simulink model "WMMSupportingForcesGP2020a"  (R2020a)
settings: Solver=ode23t  StartTime=0.0  StopTime=inf  FixedStep=.001  RelTol=1e-3  AbsTol=1e-3
InitFcn:
  | InitializeSimulationGP
  | SimulationParametersGP
values from neighbouring files (symbols this model uses):
  B11_r_B11C = [0.23805608; 0.13201777; 0]    [InitializeSimulationGP.m]
  B11_r_B11Tc1 = [L11; 0; 0]    [InitializeSimulationGP.m]
  B11_Rot_Tc1 = eye(3)    [InitializeSimulationGP.m]
  B11cI = [0.28426000 -0.06487287 0;         -0.06487287  0.54237481 0;                   0  0          0.67891020]    [InitializeSimulationGP.m]
  B12_r_B12C = [0.60504569; 0.27199376; 0.00002484]    [InitializeSimulationGP.m]
  B12_r_B12Tc2 = [L12;0;0]    [InitializeSimulationGP.m]
  B12_Rot_Tc2 = eye(3)    [InitializeSimulationGP.m]
  B12cI = [1.18803886 -2.36786418 0.00280315;          -2.36786418 6.31493281 0.00022322;           0.00280315 0.00022322 7.40915161]    [InitializeSimulationGP.m]
  B31_r_B31C = [0.35781210 0 0]    [InitializeSimulationGP.m]
  B31_Rot_B41 = eye(3)    [InitializeSimulationGP.m]
  B31cI = diag([0.03150902 0.90735702 0.90763033])    [InitializeSimulationGP.m]
  B32_r_B32C = [0.35781210 0 0]    [InitializeSimulationGP.m]
  B32_Rot_B42 = eye(3)    [InitializeSimulationGP.m]
  B32cI = diag([0.03150902 0.90735702 0.90763033])    [InitializeSimulationGP.m]
  B41_r_B41C = [0.55785997 0 0]    [InitializeSimulationGP.m]
  B41_r_B41Tc1 = [lc1;0;0]    [InitializeSimulationGP.m]
  B41cI = diag([0.00370720 0.55759812 0.55785997])    [InitializeSimulationGP.m]
  B42_r_B42C = [0.55785997 0 0]    [InitializeSimulationGP.m]
  B42_r_B42Tc2 = [lc2; 0; 0]    [InitializeSimulationGP.m]
  B42cI = diag([0.00370720 0.55759812 0.55785997])    [InitializeSimulationGP.m]
  B52_r_B52C = [0 0 0.56802906]    [InitializeSimulationGP.m]
  B52_r_B52P32 = [lc3; 0; 0]    [InitializeSimulationGP.m]
  B52_Rot_P32 = eye(3)    [InitializeSimulationGP.m]
  B52cI = diag([0.91789884, 0.91790043, 0.00091463])    [InitializeSimulationGP.m]
  Bc1_r_Bc1B11 = [L1; 0; 0]    [InitializeSimulationGP.m]
  Bc1_r_Bc1B31 = [0;0;0]    [InitializeSimulationGP.m]
  Bc1_r_Bc1C = [0.14178771; 0.16555780; 0]    [InitializeSimulationGP.m]
  Bc1_V = [0;0;0;0;0;0]    [InitializeSimulationGP.m]
  Bc1cI = [+5.892211080 +5.476111360 -0.000019630;          +5.476111360 +28.66965601 -0.000024550;          -0.000019630 -0.000024550 +29.78955950]    [InitializeSimulationGP.m]
  Bc2_r_Bc2B12 = [L2;0;0]    [InitializeSimulationGP.m]
  Bc2_r_Bc2B32 = [0;0;0]    [InitializeSimulationGP.m]
  Bc2_r_Bc2C = [0.54319901; 0.10543875; 0]    [InitializeSimulationGP.m]
  Bc2cI = [0.48071390 0.52924041 0;          0.52924041 5.80912352 0;              0      0          5.97255351]    [InitializeSimulationGP.m]
  BC_r_BCBM = [xCA; yCA; zCA]    [SimulationParametersGP.m]
  BC_Rot_BM = eye(3)    [SimulationParametersGP.m]
  BCI = diag([100 1200 1000])    [SimulationParametersGP.m]
  beta1 = atan2d(374.261,935)*pi/180    [InitializeSimulationGP.m]
  beta2 = atan2d(45.757,373.313)*pi/180    [InitializeSimulationGP.m]
  beta3 = atan2d(139.50,1132.19)*pi/180    [InitializeSimulationGP.m]
  beta4 = atan2d(88.061,296.198)*pi/180    [InitializeSimulationGP.m]
  betaGround = 1e6    (= 1000000)    [SimulationParametersGP.m]
  BFL = 0.05    [SimulationParametersGP.m]
  BFR = 0.05    [SimulationParametersGP.m]
  BM_r_BMBMp = [0;0;0]    [SimulationParametersGP.m]
  BM_Rot_BMp = [cos(gamma) -sin(gamma) 0; sin(gamma) cos(gamma) 0; 0 0 1]    [SimulationParametersGP.m]
  BMp_r_BMpBc1 = [0.185;0;0.205]    [InitializeSimulationGP.m]
  BMp_Rot_Bc1 = [cos(alpha1) -sin(alpha1)  0;                  0            0       -1;                sin(alpha1)  cos(alpha1)  0]    [InitializeSimulationGP.m]
  BRL = 0.05    [SimulationParametersGP.m]
  BRR = 0.05    [SimulationParametersGP.m]
  cc = 0.0    (= 0)    [SimulationParametersGP.m]
  D22F = [0;0;0;0;0;0]    [InitializeSimulationGP.m]
  dT = 0.01    [SimulationParametersGP.m]
  g0 = 9.8066    [SimulationParametersGP.m]
  ground_stiffness = 1e8    (= 100000000)    [SimulationParametersGP.m]
  l1 = 1.15-cc    (= 1.15)    [SimulationParametersGP.m]
  L1 = 1.0071227324212    (= 1.00712273242)    [InitializeSimulationGP.m]
  L11 = 0.37610632101293    (= 0.376106321013)    [InitializeSimulationGP.m]
  L12 = 0.30901132665325    (= 0.309011326653)    [InitializeSimulationGP.m]
  l2 = 1.15+cc    (= 1.15)    [SimulationParametersGP.m]
  L2 = 1.132185817991    (= 1.13218581799)    [InitializeSimulationGP.m]
  lc1 = 0.745    [InitializeSimulationGP.m]
  lc2 = 0.745    [InitializeSimulationGP.m]
  mB11 = 25.52660174    [InitializeSimulationGP.m]
  mB12 = 33.92850233    [InitializeSimulationGP.m]
  mB31 = 17.36281648    [InitializeSimulationGP.m]
  mB32 = 17.36281648    [InitializeSimulationGP.m]
  mB41 = 10.34519231    [InitializeSimulationGP.m]
  mB42 = 10.34519231    [InitializeSimulationGP.m]
  mB52 = 6.73059863    [InitializeSimulationGP.m]
  mBC = 2200    [SimulationParametersGP.m]
  mBc1 = 307.29601379    [InitializeSimulationGP.m]
  mBc2 = 54.58702836    [InitializeSimulationGP.m]
  mFL = 60    [SimulationParametersGP.m]
  mFR = 60    [SimulationParametersGP.m]
  mP22 = 9.26136143    [InitializeSimulationGP.m]
  mP32 = 570.18877059    [InitializeSimulationGP.m]
  mRR = 60    [SimulationParametersGP.m]
  mw = mFL    (= 60)    [SimulationParametersGP.m]
  P22_r_P22C = [0.62192523 0 0]    [InitializeSimulationGP.m]
  P22_Rot_B52 = eye(3)    [InitializeSimulationGP.m]
  P22cI = diag([0.00662754, 1.48387017, 1.48398069])    [InitializeSimulationGP.m]
  P32_r_P32C = [0.25466704; -0.13034397; -0.01302248]    [InitializeSimulationGP.m]
  P32_r_P32D22 = [0.40499744871392; -0.13130517281345; -0.013385243295654]    [InitializeSimulationGP.m]
  P32_Rot_D22 = [1 0 0;              0 0.9707729441837 0.23999977258512;              0 -0.23999977258512 0.9707729441837]    [InitializeSimulationGP.m]
  P32cI = [46.81220713 0.38607676 -0.00453819;          0.38607676 71.92201786 -1.14320993;          -0.00453819 -1.14320993 67.38128576]    [InitializeSimulationGP.m]
  R0FL = 0.35    [SimulationParametersGP.m]
  R0FR = 0.35    [SimulationParametersGP.m]
  R0RL = 0.35    [SimulationParametersGP.m]
  R0RR = 0.35    [SimulationParametersGP.m]
  Rw = R0FL    (= 0.35)    [SimulationParametersGP.m]
  Tc1_r_Tc1Bc2 = [0.098495302558553; 0.01838181329939; 0]    [InitializeSimulationGP.m]
  Tc1_Rot_Bc2 = [cos(alpha2) -sin(alpha2) 0;                sin(alpha2)  cos(alpha2) 0;                0            0           1]    [InitializeSimulationGP.m]
  Tc2_r_Tc2P22 = [-0.048858374920227;0.36587359346146;0.035276938723102]    [InitializeSimulationGP.m]
  Tc2_Rot_P22 = [0.95853460763586 -0.27664713597974  0.0683942111482;                0.28497614981675  0.93051946315663 -0.23004808784757;                0                 0.23999977258511  0.9707729441837]    [InitializeSimulationGP.m]
  Th1A = 10*pi/180    (= 0.174532925199)    [InitializeSimulationGP.m]
  Th1B = 20*pi/180    (= 0.349065850399)    [InitializeSimulationGP.m]
  Th1f = 1    [InitializeSimulationGP.m]
  Th2A = 15*pi/180    (= 0.261799387799)    [InitializeSimulationGP.m]
  Th2B = -70*pi/180    (= -1.2217304764)    [InitializeSimulationGP.m]
  Th2f = 2    [InitializeSimulationGP.m]
  w = wFL    (= 0.875)    [SimulationParametersGP.m]
  W_r_WBc1 = [0.185;0;0.205]    [InitializeSimulationGP.m]
  W_Rot_Bc1 = [cos(alpha1) -sin(alpha1)  0;                  0            0       -1;                sin(alpha1)  cos(alpha1)  0]    [InitializeSimulationGP.m]
  x10 = 0.83    [InitializeSimulationGP.m]
  x20 = 0.83    [InitializeSimulationGP.m]
  x3A = 0.2    [InitializeSimulationGP.m]
  x3B = 0.3    [InitializeSimulationGP.m]
  x3f = 1    [InitializeSimulationGP.m]
  xCA = 0.5    [SimulationParametersGP.m]
  xf = [1;0;0;0;0;0]    [InitializeSimulationGP.m]
  yCA = 0    [SimulationParametersGP.m]
  zC = 0.45    [SimulationParametersGP.m]
  zCA = .25    (= 0.25)    [SimulationParametersGP.m]
  ztau = [0;0;0;0;0;1]    [InitializeSimulationGP.m]
undefined symbols (not defined in the file or in its folder): alphaFL_meas, alphaFR_meas, alphaRL_meas, alphaRR_meas, B11_V, B11Ftot, B12_U_Tc2, B12_V, B12Ftot, B31_r_B31B41, B31_V, B31FTot, B32_r_B32B42, B32_U_B42, B32_V, B32FTot, B41_V, B41FTot, B42_Rot_Tc2, B42_U_Tc2, B42_V, B42FTot, B52_U_P32, B52_V, B52Ftot, Bc1Tot, Bc2_Rot_B12, Bc2_Rot_B32, Bc2_U_B12, Bc2_U_B32, Bc2_V, Bc2Tot, betaC_meas, D22_V, deltaFL_cmd, deltaFL_meas, deltaFR_cmd, deltaFR_meas, deltaRL_cmd, deltaRL_meas, deltaRR_cmd, deltaRR_meas, dOmegaFL_meas, dOmegaFR_meas, dOmegaRL_meas, dOmegaRR_meas, dPsi_meas, dq1, dq11, dq12, dq2, dq21, dq22, dx1, dx2, Floor, FTot_S1, FTot_S2P, FTot_S2R, FzFL ... (+63)
libraries: sm_lib x94, nesl_utility x63, simulink x5
(part 4 of 11)

== system WMMSupportingForcesGP2020a/Mobile Manipulator in Simscape/Hydraulic manipulator, Simscape ==
  note: Hydraulic manipulator in Simscape
  note: Linear hydraulic actuator forces
  Theta1 [rad] : Inport
  Theta2 [rad] : Inport  Port=2
  x3[m] : Inport  Port=3
  Base : Subsystem
      settings: PortSchema="{\"entries\":[{\"content\":{\"sides\":[{\"content\":{\"connectorIds\":[\"In1\",\"LConn1\"]},\"type\":\"ConnectorPlacement.EquallySpacedRectSide\",\"uuid\":\"74e7f3c6-cbce-4102-a556-47a2132f5eea\"},{\"content\":{\"connectorIds\":[\"RConn1\",\"RConn2\"],\"side\":\"RIGHT\"},\"type\":\"ConnectorPlacement.EquallySpacedRectSide\",\"uuid\":\"9dc74751-c8ff-4cb6-874a-dcd58e00de96\"},{\"content\":{\"connectorIds\":[\"LConn2\"],\"side\":\"TOP\"},\"type\":\"ConnectorPlacement.EquallySpacedRectSide\",\"uuid\":\"06e145de-a8a9-4531-940d-434d89c78f5b\"}]},\"type\":\"ConnectorPlacement.EquallySpacedConnector\",\"uuid\":\"f796a1f4-9531-411f-8f55-fdef488b8a52\"}],\"packageUris\":[\"http://schema.mathworks.com/mf0/Connector/R2020b\"],\"version\":\"1.0\"}"
  Bus Creator1 : BusCreator  Inputs=3
  Connection Label1 : ConnectionLabel  Label=BMp
  Connection Label11 : ConnectionLabel  Label=B12
  Connection Label12 : ConnectionLabel  Label=B52
  Connection Label14 : ConnectionLabel  Label=Bc1
  Connection Label15 : ConnectionLabel  Label=Tc2
  Connection Label16 : ConnectionLabel  Label=D22
  Connection Label29 : ConnectionLabel  Label=P22
  Connection Label3 : ConnectionLabel  Label=Tc1
  Connection Label32 : ConnectionLabel  Label=P32
  Connection Label4 : ConnectionLabel  Label=B11
  Connection Label5 : ConnectionLabel  Label=Bc2
  Connection Label6 : ConnectionLabel  Label=B31
  Connection Label7 : ConnectionLabel  Label=B42
  Connection Label8 : ConnectionLabel  Label=B32
  Connection Label9 : ConnectionLabel  Label=B41
  EndMassObject : Subsystem
      settings: PortSchema="{\"entries\":[{\"content\":{\"sides\":[{\"content\":{\"connectorIds\":[]},\"type\":\"ConnectorPlacement.EquallySpacedRectSide\",\"uuid\":\"c1652833-a888-40a4-a60e-17be9708feae\"},{\"content\":{\"connectorIds\":[],\"side\":\"RIGHT\"},\"type\":\"ConnectorPlacement.EquallySpacedRectSide\",\"uuid\":\"55671429-adc4-418e-b6f5-c624f049c776\"},{\"content\":{\"connectorIds\":[\"LConn1\",\"LConn2\"],\"side\":\"TOP\"},\"type\":\"ConnectorPlacement.EquallySpacedRectSide\",\"uuid\":\"549e793d-1b28-4f93-9706-f4524b8bc4e2\"}]},\"type\":\"ConnectorPlacement.EquallySpacedConnector\",\"uuid\":\"9a6e434f-5824-411f-a3a4-9b8ec603a501\"}],\"packageUris\":[\"http://schema.mathworks.com/mf0/Connector/R2020b\"],\"version\":\"1.0\"}"
  LiftCylinderAndLiftPiston : Subsystem
      settings: PortSchema="{\"entries\":[{\"content\":{\"sides\":[{\"content\":{\"connectorIds\":[]},\"type\":\"ConnectorPlacement.EquallySpacedRectSide\",\"uuid\":\"a609877c-275e-4024-96c6-67831631fbf9\"},{\"content\":{\"connectorIds\":[\"Out1\"],\"side\":\"RIGHT\"},\"type\":\"ConnectorPlacement.EquallySpacedRectSide\",\"uuid\":\"b747ace3-04d7-42f4-87a7-c62fd6093e0d\"},{\"content\":{\"connectorIds\":[\"LConn1\",\"LConn2\"],\"side\":\"TOP\"},\"type\":\"ConnectorPlacement.EquallySpacedRectSide\",\"uuid\":\"5f9db8d6-814e-4333-b197-0e9dcf847d3e\"},{\"content\":{\"connectorIds\":[\"RConn1\",\"RConn2\"],\"side\":\"BOTTOM\"},\"type\":\"ConnectorPlacement.EquallySpacedRectSide\",\"uuid\":\"d1d564c3-4146-4330-9936-8dd25e0cb4bf\"}]},\"type\":\"ConnectorPlacement.EquallySpacedConnector\",\"uuid\":\"d00f43c3-717c-4aa5-b919-dd57ad6708f7\"}],\"packageUris\":[\"http://schema.mathworks.com/mf0/Connector/R2020b\"],\"version\":\"1.0\"}"
  LiftLink : Subsystem
      settings: PortSchema="{\"entries\":[{\"content\":{\"sides\":[{\"content\":{\"connectorIds\":[\"LConn1\",\"LConn2\"]},\"type\":\"ConnectorPlacement.EquallySpacedRectSide\",\"uuid\":\"50668ed3-3246-41c6-a320-c5b34ebd86b6\"},{\"content\":{\"connectorIds\":[\"In1\",\"RConn1\"],\"side\":\"RIGHT\"},\"type\":\"ConnectorPlacement.EquallySpacedRectSide\",\"uuid\":\"d76ddc23-e4dc-4bdf-9e15-3eadac6cf1e2\"},{\"content\":{\"connectorIds\":[\"LConn3\"],\"side\":\"TOP\"},\"type\":\"ConnectorPlacement.EquallySpacedRectSide\",\"uuid\":\"5458eee7-805c-4d74-888c-3f811d80880c\"},{\"content\":{\"connectorIds\":[\"RConn2\",\"RConn3\",\"RConn4\"],\"side\":\"BOTTOM\"},\"type\":\"ConnectorPlacement.EquallySpacedRectSide\",\"uuid\":\"6f630415-b321-44c9-a6f9-9daa6b5086dd\"}]},\"type\":\"ConnectorPlacement.EquallySpacedConnector\",\"uuid\":\"adbb0eba-5908-47e0-8cde-3ca3a2901b66\"}],\"packageUris\":[\"http://schema.mathworks.com/mf0/Connector/R2020b\"],\"version\":\"1.0\"}"
  PrismaticJointCylinderAndPiston : Subsystem
      settings: PortSchema="{\"entries\":[{\"content\":{\"sides\":[{\"content\":{\"connectorIds\":[\"In1\"]},\"type\":\"ConnectorPlacement.EquallySpacedRectSide\",\"uuid\":\"002196eb-b81c-4ad4-9df1-33c4ef5d5c77\"},{\"content\":{\"connectorIds\":[\"Out1\"],\"side\":\"RIGHT\"},\"type\":\"ConnectorPlacement.EquallySpacedRectSide\",\"uuid\":\"e0d61efe-ea5d-4756-bea5-1d107b09975a\"},{\"content\":{\"connectorIds\":[],\"side\":\"TOP\"},\"type\":\"ConnectorPlacement.EquallySpacedRectSide\",\"uuid\":\"1a952641-c922-4f91-9854-1cf1d6e715db\"},{\"content\":{\"connectorIds\":[\"RConn1\",\"RConn2\",\"RConn3\"],\"side\":\"BOTTOM\"},\"type\":\"ConnectorPlacement.EquallySpacedRectSide\",\"uuid\":\"13c3128f-85d9-4df5-9ae2-f45a9cb5a20e\"}]},\"type\":\"ConnectorPlacement.EquallySpacedConnector\",\"uuid\":\"7bd12321-8448-494e-b8ce-fe2f63fec7f7\"}],\"packageUris\":[\"http://schema.mathworks.com/mf0/Connector/R2020b\"],\"version\":\"1.0\"}"
  TilitLink : Subsystem
      settings: PortSchema="{\"entries\":[{\"content\":{\"sides\":[{\"content\":{\"connectorIds\":[]},\"type\":\"ConnectorPlacement.EquallySpacedRectSide\",\"uuid\":\"3124f0ed-3daa-4e61-aa81-877c0a0fd3a0\"},{\"content\":{\"connectorIds\":[\"RConn1\"],\"side\":\"RIGHT\"},\"type\":\"ConnectorPlacement.EquallySpacedRectSide\",\"uuid\":\"bc27bd78-7de5-476c-8b4b-17e2ed4c2476\"},{\"content\":{\"connectorIds\":[\"LConn1\",\"LConn2\",\"LConn3\",\"LConn4\"],\"side\":\"TOP\"},\"type\":\"ConnectorPlacement.EquallySpacedRectSide\",\"uuid\":\"46b542cf-bb62-4410-9418-b726c84ee3f9\"}]},\"type\":\"ConnectorPlacement.EquallySpacedConnector\",\"uuid\":\"3938a7f2-fa69-42c9-abcf-1c8c25e9b66f\"}],\"packageUris\":[\"http://schema.mathworks.com/mf0/Connector/R2020b\"],\"version\":\"1.0\"}"
  TiltCylinderAndTiltPiston : Subsystem
      settings: PortSchema="{\"entries\":[{\"content\":{\"sides\":[{\"content\":{\"connectorIds\":[]},\"type\":\"ConnectorPlacement.EquallySpacedRectSide\",\"uuid\":\"a609877c-275e-4024-96c6-67831631fbf9\"},{\"content\":{\"connectorIds\":[\"Out1\"],\"side\":\"RIGHT\"},\"type\":\"ConnectorPlacement.EquallySpacedRectSide\",\"uuid\":\"b747ace3-04d7-42f4-87a7-c62fd6093e0d\"},{\"content\":{\"connectorIds\":[\"LConn1\",\"LConn2\"],\"side\":\"TOP\"},\"type\":\"ConnectorPlacement.EquallySpacedRectSide\",\"uuid\":\"5f9db8d6-814e-4333-b197-0e9dcf847d3e\"},{\"content\":{\"connectorIds\":[\"RConn1\",\"RConn2\"],\"side\":\"BOTTOM\"},\"type\":\"ConnectorPlacement.EquallySpacedRectSide\",\"uuid\":\"d1d564c3-4146-4330-9936-8dd25e0cb4bf\"}]},\"type\":\"ConnectorPlacement.EquallySpacedConnector\",\"uuid\":\"d00f43c3-717c-4aa5-b919-dd57ad6708f7\"}],\"packageUris\":[\"http://schema.mathworks.com/mf0/Connector/R2020b\"],\"version\":\"1.0\"}"
  BMp : PMIOPort  Side=Left
  fcx_SS : Outport
  wires:
  LiftCylinderAndLiftPiston/1(fc1) -> [fc1]
  TiltCylinderAndTiltPiston/1(fc2) -> [fc2]
  x3[m]/1 -> PrismaticJointCylinderAndPiston/1(x3)
  PrismaticJointCylinderAndPiston/1(fc3) -> [fc3]
  Theta1 [rad]/1 -> Base/1(Theta1[rad])
  Theta2 [rad]/1 -> LiftLink/1(Theta2[rad])
  [fc1] -> Bus Creator1/1  "fc1_SS"
  [fc2] -> Bus Creator1/2  "fc2_SS"
  [fc3] -> Bus Creator1/3  "fc3_SS"
  Bus Creator1/1 -> fcx_SS/1
  connections:
  BMp/RConn1 -- Base/LConn1 -- Connection Label1/LConn1
  LiftLink/LConn1 -- TiltCylinderAndTiltPiston/RConn1
  LiftLink/LConn2 -- TilitLink/RConn1
  TiltCylinderAndTiltPiston/RConn2 -- TilitLink/LConn4
  LiftCylinderAndLiftPiston/RConn2 -- LiftLink/LConn3
  Base/RConn2 -- LiftLink/RConn1
  LiftCylinderAndLiftPiston/RConn1 -- Base/RConn1
  LiftLink/RConn4 -- Connection Label3/LConn1
  Connection Label4/LConn1 -- LiftLink/RConn3
  Connection Label5/LConn1 -- LiftLink/RConn2
  Connection Label6/LConn1 -- LiftCylinderAndLiftPiston/LConn1
  Connection Label9/LConn1 -- LiftCylinderAndLiftPiston/LConn2
  Connection Label7/LConn1 -- TiltCylinderAndTiltPiston/LConn2
  Connection Label8/LConn1 -- TiltCylinderAndTiltPiston/LConn1
  Connection Label11/LConn1 -- TilitLink/LConn3
  Connection Label15/LConn1 -- TilitLink/LConn2
  Connection Label16/LConn1 -- EndMassObject/LConn2
  Connection Label14/LConn1 -- Base/LConn2
  Connection Label12/LConn1 -- PrismaticJointCylinderAndPiston/RConn3
  PrismaticJointCylinderAndPiston/RConn1 -- Connection Label29/LConn1 -- TilitLink/LConn1
  PrismaticJointCylinderAndPiston/RConn2 -- EndMassObject/LConn1 -- Connection Label32/LConn1

== system WMMSupportingForcesGP2020a/Mobile Manipulator in Simscape/SteeringFL ==
  deltaFL_cmd : Inport
  PS-Simulink Converter : nesl_utility/PS-Simulink Converter  PhysicalDomain=network_engine_domain  SubClassName=ps_output  LeftPortType=input  RightPortType=output  PseudoPeriodic=off  Frequencies=[]  Unit=inherit  AffineConversion=off
      settings: SourceProductBaseCode=PW,SS
  Revolute Joint2 : sm_lib/Joints/Revolute Joint  JointMode=Normal  SenseConstraintForce=off  SenseConstraintForceX=off  SenseConstraintForceY=off  SenseConstraintForceZ=off  SenseConstraintTorque=off  SenseConstraintTorqueX=off  SenseConstraintTorqueY=off  SenseConstraintTorqueZ=off  SenseTotalForce=off  SenseTotalForceX=off  SenseTotalForceY=off  SenseTotalForceZ=off  SenseTotalTorque=off  SenseTotalTorqueX=off  SenseTotalTorqueY=off  SenseTotalTorqueZ=off  CompositeWrenchDir=FollowerOnBase  CompositeWrenchFrame=BaseFrame  EquilibriumPosition=0  EquilibriumPositionUnits=rad  SpringStiffness=0  SpringStiffnessUnits=N*m/rad  DampingCoefficient=.0001  DampingCoefficientUnits=N*m/(rad/s)  TorqueActuationMode=ComputedTorque  MotionActuationMode=InputMotion  SensePosition=on  SenseVelocity=off  SenseAcceleration=off  SenseTorqueForce=off  SenseLowerLimitTorqueForce=off  SenseUpperLimitTorqueForce=off  LowerLimitSpecify=off  LowerLimitBound=-90  LowerLimitBoundUnits=deg  LowerLimitStiffness=1e4  LowerLimitStiffnessUnits=N*m/deg  LowerLimitDamping=10  LowerLimitDampingUnits=N*m/(deg/s)  LowerLimitTransitionRegionWidth=0.1  LowerLimitTransitionRegionWidthUnits=deg  UpperLimitSpecify=off  UpperLimitBound=90  UpperLimitBoundUnits=deg  UpperLimitStiffness=1e4  UpperLimitStiffnessUnits=N*m/deg  UpperLimitDamping=10  UpperLimitDampingUnits=N*m/(deg/s)  UpperLimitTransitionRegionWidth=0.1  UpperLimitTransitionRegionWidthUnits=deg  PositionTargetSpecify=off  PositionTargetPriority=High  PositionTargetValue=0  PositionTargetValueUnits=deg  VelocityTargetSpecify=off  VelocityTargetPriority=High  VelocityTargetValue=0  VelocityTargetValueUnits=deg/s
  Simulink-PS Converter7 : nesl_utility/Simulink-PS Converter  PhysicalDomain=network_engine_domain  SubClassName=ps_input  LeftPortType=input  RightPortType=output  PseudoPeriodic=off  Frequencies=[]  NoiseDistribution=none  NoiseParameters=[]  Unit=rad  AffineConversion=off  FilteringAndDerivatives=filter  SimscapeFilterOrder=2  InputFilterTimeConstant=0.001  UdotUserProvided=0
      settings: SourceProductBaseCode=PW,SS
  WFL : PMIOPort  Side=Left
  CFL : PMIOPort  Port=2  Side=Right
  deltaFL_meas : Outport
  wires:
  deltaFL_cmd/1 -> Simulink-PS Converter7/1
  PS-Simulink Converter/1 -> deltaFL_meas/1
  connections:
  Simulink-PS Converter7/RConn1 -- Revolute Joint2/LConn2
  Revolute Joint2/LConn1 -- CFL/RConn1
  Revolute Joint2/RConn1 -- WFL/RConn1
  PS-Simulink Converter/LConn1 -- Revolute Joint2/RConn2

== system WMMSupportingForcesGP2020a/Mobile Manipulator in Simscape/SteeringFR ==
  deltaFR_cmd : Inport
  PS-Simulink Converter : nesl_utility/PS-Simulink Converter  PhysicalDomain=network_engine_domain  SubClassName=ps_output  LeftPortType=input  RightPortType=output  PseudoPeriodic=off  Frequencies=[]  Unit=inherit  AffineConversion=off
      settings: SourceProductBaseCode=PW,SS
  Revolute Joint2 : sm_lib/Joints/Revolute Joint  JointMode=Normal  SenseConstraintForce=off  SenseConstraintForceX=off  SenseConstraintForceY=off  SenseConstraintForceZ=off  SenseConstraintTorque=off  SenseConstraintTorqueX=off  SenseConstraintTorqueY=off  SenseConstraintTorqueZ=off  SenseTotalForce=off  SenseTotalForceX=off  SenseTotalForceY=off  SenseTotalForceZ=off  SenseTotalTorque=off  SenseTotalTorqueX=off  SenseTotalTorqueY=off  SenseTotalTorqueZ=off  CompositeWrenchDir=FollowerOnBase  CompositeWrenchFrame=BaseFrame  EquilibriumPosition=0  EquilibriumPositionUnits=rad  SpringStiffness=0  SpringStiffnessUnits=N*m/rad  DampingCoefficient=.0001  DampingCoefficientUnits=N*m/(rad/s)  TorqueActuationMode=ComputedTorque  MotionActuationMode=InputMotion  SensePosition=on  SenseVelocity=off  SenseAcceleration=off  SenseTorqueForce=off  SenseLowerLimitTorqueForce=off  SenseUpperLimitTorqueForce=off  LowerLimitSpecify=off  LowerLimitBound=-90  LowerLimitBoundUnits=deg  LowerLimitStiffness=1e4  LowerLimitStiffnessUnits=N*m/deg  LowerLimitDamping=10  LowerLimitDampingUnits=N*m/(deg/s)  LowerLimitTransitionRegionWidth=0.1  LowerLimitTransitionRegionWidthUnits=deg  UpperLimitSpecify=off  UpperLimitBound=90  UpperLimitBoundUnits=deg  UpperLimitStiffness=1e4  UpperLimitStiffnessUnits=N*m/deg  UpperLimitDamping=10  UpperLimitDampingUnits=N*m/(deg/s)  UpperLimitTransitionRegionWidth=0.1  UpperLimitTransitionRegionWidthUnits=deg  PositionTargetSpecify=off  PositionTargetPriority=High  PositionTargetValue=0  PositionTargetValueUnits=deg  VelocityTargetSpecify=off  VelocityTargetPriority=High  VelocityTargetValue=0  VelocityTargetValueUnits=deg/s
  Simulink-PS Converter7 : nesl_utility/Simulink-PS Converter  PhysicalDomain=network_engine_domain  SubClassName=ps_input  LeftPortType=input  RightPortType=output  PseudoPeriodic=off  Frequencies=[]  NoiseDistribution=none  NoiseParameters=[]  Unit=rad  AffineConversion=off  FilteringAndDerivatives=filter  SimscapeFilterOrder=2  InputFilterTimeConstant=0.001  UdotUserProvided=0
      settings: SourceProductBaseCode=PW,SS
  WFR : PMIOPort  Side=Left
  CFR : PMIOPort  Port=2  Side=Right
  deltaFR_meas : Outport
  wires:
  deltaFR_cmd/1 -> Simulink-PS Converter7/1
  PS-Simulink Converter/1 -> deltaFR_meas/1
  connections:
  Simulink-PS Converter7/RConn1 -- Revolute Joint2/LConn2
  Revolute Joint2/LConn1 -- CFR/RConn1
  Revolute Joint2/RConn1 -- WFR/RConn1
  PS-Simulink Converter/LConn1 -- Revolute Joint2/RConn2

== system WMMSupportingForcesGP2020a/Mobile Manipulator in Simscape/SteeringRL ==
  deltaRL_cmd : Inport
  PS-Simulink Converter : nesl_utility/PS-Simulink Converter  PhysicalDomain=network_engine_domain  SubClassName=ps_output  LeftPortType=input  RightPortType=output  PseudoPeriodic=off  Frequencies=[]  Unit=inherit  AffineConversion=off
      settings: SourceProductBaseCode=PW,SS
  Revolute Joint2 : sm_lib/Joints/Revolute Joint  JointMode=Normal  SenseConstraintForce=off  SenseConstraintForceX=off  SenseConstraintForceY=off  SenseConstraintForceZ=off  SenseConstraintTorque=off  SenseConstraintTorqueX=off  SenseConstraintTorqueY=off  SenseConstraintTorqueZ=off  SenseTotalForce=off  SenseTotalForceX=off  SenseTotalForceY=off  SenseTotalForceZ=off  SenseTotalTorque=off  SenseTotalTorqueX=off  SenseTotalTorqueY=off  SenseTotalTorqueZ=off  CompositeWrenchDir=FollowerOnBase  CompositeWrenchFrame=BaseFrame  EquilibriumPosition=0  EquilibriumPositionUnits=deg  SpringStiffness=0  SpringStiffnessUnits=N*m/deg  DampingCoefficient=.0001  DampingCoefficientUnits=N*m/(deg/s)  TorqueActuationMode=ComputedTorque  MotionActuationMode=InputMotion  SensePosition=on  SenseVelocity=off  SenseAcceleration=off  SenseTorqueForce=off  SenseLowerLimitTorqueForce=off  SenseUpperLimitTorqueForce=off  LowerLimitSpecify=off  LowerLimitBound=-90  LowerLimitBoundUnits=deg  LowerLimitStiffness=1e4  LowerLimitStiffnessUnits=N*m/deg  LowerLimitDamping=10  LowerLimitDampingUnits=N*m/(deg/s)  LowerLimitTransitionRegionWidth=0.1  LowerLimitTransitionRegionWidthUnits=deg  UpperLimitSpecify=off  UpperLimitBound=90  UpperLimitBoundUnits=deg  UpperLimitStiffness=1e4  UpperLimitStiffnessUnits=N*m/deg  UpperLimitDamping=10  UpperLimitDampingUnits=N*m/(deg/s)  UpperLimitTransitionRegionWidth=0.1  UpperLimitTransitionRegionWidthUnits=deg  PositionTargetSpecify=off  PositionTargetPriority=High  PositionTargetValue=0  PositionTargetValueUnits=deg  VelocityTargetSpecify=off  VelocityTargetPriority=High  VelocityTargetValue=0  VelocityTargetValueUnits=deg/s
  Simulink-PS Converter7 : nesl_utility/Simulink-PS Converter  PhysicalDomain=network_engine_domain  SubClassName=ps_input  LeftPortType=input  RightPortType=output  PseudoPeriodic=off  Frequencies=[]  NoiseDistribution=none  NoiseParameters=[]  Unit=rad  AffineConversion=off  FilteringAndDerivatives=filter  SimscapeFilterOrder=2  InputFilterTimeConstant=0.001  UdotUserProvided=0
      settings: SourceProductBaseCode=PW,SS
  WRL : PMIOPort  Side=Left
  CRL : PMIOPort  Port=2  Side=Right
  deltaRL_meas : Outport
  wires:
  deltaRL_cmd/1 -> Simulink-PS Converter7/1
  PS-Simulink Converter/1 -> deltaRL_meas/1
  connections:
  Simulink-PS Converter7/RConn1 -- Revolute Joint2/LConn2
  Revolute Joint2/LConn1 -- CRL/RConn1
  Revolute Joint2/RConn1 -- WRL/RConn1
  PS-Simulink Converter/LConn1 -- Revolute Joint2/RConn2

== system WMMSupportingForcesGP2020a/Mobile Manipulator in Simscape/SteeringRR ==
  deltaRR_cmd : Inport
  PS-Simulink Converter : nesl_utility/PS-Simulink Converter  PhysicalDomain=network_engine_domain  SubClassName=ps_output  LeftPortType=input  RightPortType=output  PseudoPeriodic=off  Frequencies=[]  Unit=inherit  AffineConversion=off
      settings: SourceProductBaseCode=PW,SS
  Revolute Joint2 : sm_lib/Joints/Revolute Joint  JointMode=Normal  SenseConstraintForce=off  SenseConstraintForceX=off  SenseConstraintForceY=off  SenseConstraintForceZ=off  SenseConstraintTorque=off  SenseConstraintTorqueX=off  SenseConstraintTorqueY=off  SenseConstraintTorqueZ=off  SenseTotalForce=off  SenseTotalForceX=off  SenseTotalForceY=off  SenseTotalForceZ=off  SenseTotalTorque=off  SenseTotalTorqueX=off  SenseTotalTorqueY=off  SenseTotalTorqueZ=off  CompositeWrenchDir=FollowerOnBase  CompositeWrenchFrame=BaseFrame  EquilibriumPosition=0  EquilibriumPositionUnits=deg  SpringStiffness=0  SpringStiffnessUnits=N*m/deg  DampingCoefficient=.0001  DampingCoefficientUnits=N*m/(deg/s)  TorqueActuationMode=ComputedTorque  MotionActuationMode=InputMotion  SensePosition=on  SenseVelocity=off  SenseAcceleration=off  SenseTorqueForce=off  SenseLowerLimitTorqueForce=off  SenseUpperLimitTorqueForce=off  LowerLimitSpecify=off  LowerLimitBound=-90  LowerLimitBoundUnits=deg  LowerLimitStiffness=1e4  LowerLimitStiffnessUnits=N*m/deg  LowerLimitDamping=10  LowerLimitDampingUnits=N*m/(deg/s)  LowerLimitTransitionRegionWidth=0.1  LowerLimitTransitionRegionWidthUnits=deg  UpperLimitSpecify=off  UpperLimitBound=90  UpperLimitBoundUnits=deg  UpperLimitStiffness=1e4  UpperLimitStiffnessUnits=N*m/deg  UpperLimitDamping=10  UpperLimitDampingUnits=N*m/(deg/s)  UpperLimitTransitionRegionWidth=0.1  UpperLimitTransitionRegionWidthUnits=deg  PositionTargetSpecify=off  PositionTargetPriority=High  PositionTargetValue=0  PositionTargetValueUnits=deg  VelocityTargetSpecify=off  VelocityTargetPriority=High  VelocityTargetValue=0  VelocityTargetValueUnits=deg/s
  Simulink-PS Converter7 : nesl_utility/Simulink-PS Converter  PhysicalDomain=network_engine_domain  SubClassName=ps_input  LeftPortType=input  RightPortType=output  PseudoPeriodic=off  Frequencies=[]  NoiseDistribution=none  NoiseParameters=[]  Unit=rad  AffineConversion=off  FilteringAndDerivatives=filter  SimscapeFilterOrder=2  InputFilterTimeConstant=0.001  UdotUserProvided=0
      settings: SourceProductBaseCode=PW,SS
  WRR : PMIOPort  Side=Left
  CRR : PMIOPort  Port=2  Side=Right
  deltaRR_meas : Outport
  wires:
  deltaRR_cmd/1 -> Simulink-PS Converter7/1
  PS-Simulink Converter/1 -> deltaRR_meas/1
  connections:
  Simulink-PS Converter7/RConn1 -- Revolute Joint2/LConn2
  Revolute Joint2/LConn1 -- CRR/RConn1
  Revolute Joint2/RConn1 -- WRR/RConn1
  PS-Simulink Converter/LConn1 -- Revolute Joint2/RConn2

== system WMMSupportingForcesGP2020a/Mobile Manipulator in Simscape/Subsystem ==
  File Solid1 : sm_lib/Body Elements/File Solid  ExtGeomFileName=Wheel.STEP  UnitType=FromFile  ExtGeomFileUnits=m  StepReaderType=HEX  ExportConvexHullGeometry=off  InertiaType=CalculateFromGeometry  Mass=mFL  MassUnits=kg  CenterOfMass=[0 0 0]  CenterOfMassUnits=m  MomentsOfInertia=[1 1 1]  MomentsOfInertiaUnits=kg*m^2  ProductsOfInertia=[0 0 0]  ProductsOfInertiaUnits=kg*m^2  BasedOnType=Mass  Density=200  DensityUnits=kg/m^3  DoExposeReferenceFrame=off  SerializedFrames=<Frames><Frame><Id>Frame1</Id><Value><Name>WFLp</Name><Origin><Source>ReferenceFrame</Source><FeatureName></FeatureName></Origin><PrimaryAxis><DefinedDirection>+Z</DefinedDirection><Source>ReferenceFrame</Source><SourceDirection>+Z</SourceDirection><FeatureName></FeatureName></PrimaryAxis><SecondaryAxis><DefinedDirection>+X</DefinedDirection><Source>ReferenceFrame</Source><SourceDirection>+X</SourceDirection><FeatureName></FeatureName></SecondaryAxis></Value></Frame></Frames>  GraphicType=FromGeometry  MarkerShape=Sphere  MarkerSize=10  GraphicVisPropType=SimpleVisualProperties  GraphicDiffuseColor=[0.8 0.6 0.0]  GraphicSpecularColor=[0.5 0.5 0.5 1.0]  GraphicAmbientColor=[0.15 0.15 0.15 1.0]  GraphicEmissiveColor=[0.0 0.0 0.0 1.0]  GraphicShininess=75  GraphicOpacity=1.0
  WFLp : PMIOPort  Side=Left
  connections:
  WFLp/RConn1 -- File Solid1/LConn1

== system WMMSupportingForcesGP2020a/Mobile Manipulator in Simscape/Subsystem6 ==
  File Solid3 : sm_lib/Body Elements/File Solid  ExtGeomFileName=Wheel.STEP  UnitType=FromFile  ExtGeomFileUnits=m  StepReaderType=HEX  ExportConvexHullGeometry=off  InertiaType=CalculateFromGeometry  Mass=mFR  MassUnits=kg  CenterOfMass=[0 0 0]  CenterOfMassUnits=m  MomentsOfInertia=[1 1 1]  MomentsOfInertiaUnits=kg*m^2  ProductsOfInertia=[0 0 0]  ProductsOfInertiaUnits=kg*m^2  BasedOnType=Mass  Density=200  DensityUnits=kg/m^3  DoExposeReferenceFrame=off  SerializedFrames=<Frames><Frame><Id>Frame1</Id><Value><Name>WRL</Name><Origin><Source>ReferenceFrame</Source><FeatureName></FeatureName></Origin><PrimaryAxis><DefinedDirection>+Z</DefinedDirection><Source>ReferenceFrame</Source><SourceDirection>+Z</SourceDirection><FeatureName></FeatureName></PrimaryAxis><SecondaryAxis><DefinedDirection>+X</DefinedDirection><Source>ReferenceFrame</Source><SourceDirection>+X</SourceDirection><FeatureName></FeatureName></SecondaryAxis></Value></Frame></Frames>  GraphicType=FromGeometry  MarkerShape=Sphere  MarkerSize=10  GraphicVisPropType=SimpleVisualProperties  GraphicDiffuseColor=[0.8 0.6 0.0]  GraphicSpecularColor=[0.5 0.5 0.5 1.0]  GraphicAmbientColor=[0.15 0.15 0.15 1.0]  GraphicEmissiveColor=[0.0 0.0 0.0 1.0]  GraphicShininess=75  GraphicOpacity=1.0
  WRLp : PMIOPort  Side=Left
  connections:
  File Solid3/LConn1 -- WRLp/RConn1

== system WMMSupportingForcesGP2020a/Mobile Manipulator in Simscape/Subsystem7 ==
  File Solid2 : sm_lib/Body Elements/File Solid  ExtGeomFileName=Wheel.STEP  UnitType=FromFile  ExtGeomFileUnits=m  StepReaderType=HEX  ExportConvexHullGeometry=off  InertiaType=CalculateFromGeometry  Mass=mRR  MassUnits=kg  CenterOfMass=[0 0 0]  CenterOfMassUnits=m  MomentsOfInertia=[1 1 1]  MomentsOfInertiaUnits=kg*m^2  ProductsOfInertia=[0 0 0]  ProductsOfInertiaUnits=kg*m^2  BasedOnType=Mass  Density=200  DensityUnits=kg/m^3  DoExposeReferenceFrame=off  SerializedFrames=<Frames><Frame><Id>Frame1</Id><Value><Name>WRRp</Name><Origin><Source>ReferenceFrame</Source><FeatureName></FeatureName></Origin><PrimaryAxis><DefinedDirection>+Z</DefinedDirection><Source>ReferenceFrame</Source><SourceDirection>+Z</SourceDirection><FeatureName></FeatureName></PrimaryAxis><SecondaryAxis><DefinedDirection>+X</DefinedDirection><Source>ReferenceFrame</Source><SourceDirection>-X</SourceDirection><FeatureName></FeatureName></SecondaryAxis></Value></Frame></Frames>  GraphicType=FromGeometry  MarkerShape=Sphere  MarkerSize=10  GraphicVisPropType=SimpleVisualProperties  GraphicDiffuseColor=[0.8 0.6 0.0]  GraphicSpecularColor=[0.5 0.5 0.5 1.0]  GraphicAmbientColor=[0.15 0.15 0.15 1.0]  GraphicEmissiveColor=[0.0 0.0 0.0 1.0]  GraphicShininess=75  GraphicOpacity=1.0
  WRRp : PMIOPort  Side=Left
  connections:
  File Solid2/LConn1 -- WRRp/RConn1

== system WMMSupportingForcesGP2020a/Mobile Manipulator in Simscape/Subsystem8 ==
  File Solid4 : sm_lib/Body Elements/File Solid  ExtGeomFileName=Wheel.STEP  UnitType=FromFile  ExtGeomFileUnits=m  StepReaderType=HEX  ExportConvexHullGeometry=off  InertiaType=CalculateFromGeometry  Mass=mFR  MassUnits=kg  CenterOfMass=[0 0 0]  CenterOfMassUnits=m  MomentsOfInertia=[1 1 1]  MomentsOfInertiaUnits=kg*m^2  ProductsOfInertia=[0 0 0]  ProductsOfInertiaUnits=kg*m^2  BasedOnType=Mass  Density=200  DensityUnits=kg/m^3  DoExposeReferenceFrame=off  SerializedFrames=<Frames><Frame><Id>Frame1</Id><Value><Name>WFRp</Name><Origin><Source>ReferenceFrame</Source><FeatureName></FeatureName></Origin><PrimaryAxis><DefinedDirection>+Z</DefinedDirection><Source>ReferenceFrame</Source><SourceDirection>+Z</SourceDirection><FeatureName></FeatureName></PrimaryAxis><SecondaryAxis><DefinedDirection>+X</DefinedDirection><Source>ReferenceFrame</Source><SourceDirection>-X</SourceDirection><FeatureName></FeatureName></SecondaryAxis></Value></Frame></Frames>  GraphicType=FromGeometry  MarkerShape=Sphere  MarkerSize=10  GraphicVisPropType=SimpleVisualProperties  GraphicDiffuseColor=[0.8 0.6 0.0]  GraphicSpecularColor=[0.5 0.5 0.5 1.0]  GraphicAmbientColor=[0.15 0.15 0.15 1.0]  GraphicEmissiveColor=[0.0 0.0 0.0 1.0]  GraphicShininess=75  GraphicOpacity=1.0
  WFRp : PMIOPort  Side=Left
  connections:
  WFRp/RConn1 -- File Solid4/LConn1

== system WMMSupportingForcesGP2020a/Mobile Manipulator in Simscape/WFL_kinematic_quantities ==
  note: Friction momemnt and more to be added.
  FzFL_meas : Inport
  FL_kin : Inport  Port=2
  MyaFL : Inport  Port=3
  Bus Selector : BusSelector  OutputSignals=alphaFL_meas,dOmegaFL_meas,kappaFL_meas,ReFL,VxFL_meas
  Constant : Constant  Value=0
  External Force and Torque1 : sm_lib/Forces and Torques/External Force and Torque  ForceResolutionFrame=AttachedFrame  EnableForceX=off  EnableForceY=off  EnableForceZ=off  EnableForce=off  TorqueResolutionFrame=AttachedFrame  EnableTorqueX=off  EnableTorqueY=on  EnableTorqueZ=off  EnableTorque=off
  External Force and Torque5 : sm_lib/Forces and Torques/External Force and Torque  ForceResolutionFrame=AttachedFrame  EnableForceX=on  EnableForceY=on  EnableForceZ=on  EnableForce=off  TorqueResolutionFrame=AttachedFrame  EnableTorqueX=on  EnableTorqueY=on  EnableTorqueZ=off  EnableTorque=off
  Gain4 : Gain  Gain=R0FL
  Gain5 : Gain  Gain=-R0FL
  Gain6 : Gain  Gain=1e4
  Product : Product
  Product2 : Product
  Simulink-PS Converter{1..3,7,11,13} (6 alike) : nesl_utility/Simulink-PS Converter  PhysicalDomain=network_engine_domain  SubClassName=ps_input  LeftPortType=input  RightPortType=output  PseudoPeriodic=off  Frequencies=[]  NoiseDistribution=none  NoiseParameters=[]  Unit=1  AffineConversion=off  FilteringAndDerivatives=provide  SimscapeFilterOrder=1  InputFilterTimeConstant=0.001  UdotUserProvided=0
      settings: SourceProductBaseCode=PW,SS
  Sum2 : Sum  Inputs=-++
  Tanh : Trigonometry  Operator=tanh
  Terminator : Terminator
  lateralForceFL : MATLAB Function  TreatAsAtomicUnit=on
  longitudinalForceFL : MATLAB Function  TreatAsAtomicUnit=on
  WFL : PMIOPort  Side=Left
  WFLp : PMIOPort  Port=2  Side=Left
  wires:
  [ReFL] -> Product/1
  [FzFL_meas] -> Simulink-PS Converter7/1
  [FzFL_meas] -> lateralForceFL/1(FzFL)
  Bus Selector/1 -> [alphaFL_meas]  "<alphaFL_meas>"
  [FzFL_meas] -> longitudinalForceFL/1(FzFL)
  Bus Selector/4 -> [ReFL]  "<ReFL>"
  Bus Selector/3 -> [kappaFL_meas]  "<kappaFL_meas>"
  Bus Selector/2 -> Terminator/1  "<dOmegaFL_meas>"
  FzFL_meas/1 -> [FzFL_meas]
  FL_kin/1 -> Bus Selector/1
  Sum2/1 -> Simulink-PS Converter2/1
  [FxFL] -> Product/2
  [MyaFL] -> Sum2/3
  [FxFL] -> Simulink-PS Converter13/1
  Product/1 -> Sum2/1
  Constant/1 -> Sum2/2
  [FyFL] -> Simulink-PS Converter11/1
  [FxFL] -> Gain5/1
  Gain5/1 -> Simulink-PS Converter3/1
  [FyFL] -> Gain4/1
  Gain4/1 -> Simulink-PS Converter1/1
  MyaFL/1 -> [MyaFL]
  Bus Selector/5 -> [VxFL_meas]  "<VxFL_meas>"
  lateralForceFL/1(FyFL) -> [FyFL]
  longitudinalForceFL/1(FxFL) -> Product2/2
  Product2/1 -> [FxFL]
  [sgnVxFL] -> Product2/1
  [kappaFL_meas] -> longitudinalForceFL/2(kappaFL)
  [alphaFL_meas] -> lateralForceFL/2(alphaFL)
  Tanh/1 -> [sgnVxFL]
  Gain6/1 -> Tanh/1
  [VxFL_meas] -> Gain6/1
  connections:
  Simulink-PS Converter2/RConn1 -- External Force and Torque1/LConn1
  Simulink-PS Converter11/RConn1 -- External Force and Torque5/LConn2
  Simulink-PS Converter7/RConn1 -- External Force and Torque5/LConn3
  External Force and Torque1/RConn1 -- WFLp/RConn1
  Simulink-PS Converter13/RConn1 -- External Force and Torque5/LConn1
  External Force and Torque5/RConn1 -- WFL/RConn1
  Simulink-PS Converter1/RConn1 -- External Force and Torque5/LConn4
  Simulink-PS Converter3/RConn1 -- External Force and Torque5/LConn5

== system WMMSupportingForcesGP2020a/Mobile Manipulator in Simscape/WFR_kinematic_quantities ==
  note: Friction momemnt and more to be added.
  FzFR_meas : Inport
  FR_kin : Inport  Port=2
  MyaFR : Inport  Port=3
  Bus Selector : BusSelector  OutputSignals=alphaFR_meas,dOmegaFR_meas,kappaFR_meas,ReFR,VxFR_meas
  Constant : Constant  Value=0
  External Force and Torque1 : sm_lib/Forces and Torques/External Force and Torque  ForceResolutionFrame=AttachedFrame  EnableForceX=off  EnableForceY=off  EnableForceZ=off  EnableForce=off  TorqueResolutionFrame=AttachedFrame  EnableTorqueX=off  EnableTorqueY=on  EnableTorqueZ=off  EnableTorque=off
  External Force and Torque5 : sm_lib/Forces and Torques/External Force and Torque  ForceResolutionFrame=AttachedFrame  EnableForceX=on  EnableForceY=on  EnableForceZ=on  EnableForce=off  TorqueResolutionFrame=AttachedFrame  EnableTorqueX=on  EnableTorqueY=on  EnableTorqueZ=off  EnableTorque=off
  Gain : Gain  Gain=1e4
  Gain5 : Gain  Gain=R0FR
  Gain6 : Gain  Gain=-R0FR
  Product : Product
  Product2 : Product
  Simulink-PS Converter{1..3,7,11,13} (6 alike) : nesl_utility/Simulink-PS Converter  PhysicalDomain=network_engine_domain  SubClassName=ps_input  LeftPortType=input  RightPortType=output  PseudoPeriodic=off  Frequencies=[]  NoiseDistribution=none  NoiseParameters=[]  Unit=1  AffineConversion=off  FilteringAndDerivatives=provide  SimscapeFilterOrder=1  InputFilterTimeConstant=0.001  UdotUserProvided=0
      settings: SourceProductBaseCode=PW,SS
  Sum2 : Sum  Inputs=-++
  Tanh : Trigonometry  Operator=tanh
  Terminator : Terminator
  lateralForceFR : MATLAB Function  TreatAsAtomicUnit=on
  longitudinalForceFR : MATLAB Function  TreatAsAtomicUnit=on
  WFR : PMIOPort  Side=Left
  WFRp : PMIOPort  Port=2  Side=Left
  wires:
  [MyaFR] -> Sum2/3
  [FxFR] -> Product/2
  Sum2/1 -> Simulink-PS Converter2/1
  FR_kin/1 -> Bus Selector/1
  FzFR_meas/1 -> [FzFR_meas]
  Bus Selector/2 -> Terminator/1  "<dOmegaFR_meas>"
  Bus Selector/3 -> [kappaFR_meas]  "<kappaFR_meas>"
  Bus Selector/4 -> [ReFR]  "<ReFR>"
  [FzFR_meas] -> longitudinalForceFR/1(FzFR)
  Bus Selector/1 -> [alphaFR_meas]  "<alphaFR_meas>"
  [FzFR_meas] -> lateralForceFR/1(FzFR)
  [ReFR] -> Product/1
  MyaFR/1 -> [MyaFR]
  [FxFR] -> Simulink-PS Converter13/1
  [FyFR] -> Simulink-PS Converter11/1
  [FzFR_meas] -> Simulink-PS Converter7/1
  Product/1 -> Sum2/1
  Gain6/1 -> Simulink-PS Converter3/1
  Gain5/1 -> Simulink-PS Converter1/1
  [FxFR] -> Gain6/1
  [FyFR] -> Gain5/1
  Bus Selector/5 -> [VxFR_meas]  "<VxFR_meas>"
  lateralForceFR/1(FyFR) -> [FyFR]
  Product2/1 -> [FxFR]
  longitudinalForceFR/1(FxFR) -> Product2/2
  [sgnVxFR] -> Product2/1
  [kappaFR_meas] -> longitudinalForceFR/2(kappaFR)
  [alphaFR_meas] -> lateralForceFR/2(alphaFR)
  [VxFR_meas] -> Gain/1
  Tanh/1 -> [sgnVxFR]
  Gain/1 -> Tanh/1
  Constant/1 -> Sum2/2
  connections:
  Simulink-PS Converter13/RConn1 -- External Force and Torque5/LConn1
  External Force and Torque1/RConn1 -- WFRp/RConn1
  Simulink-PS Converter7/RConn1 -- External Force and Torque5/LConn3
  Simulink-PS Converter11/RConn1 -- External Force and Torque5/LConn2
  Simulink-PS Converter2/RConn1 -- External Force and Torque1/LConn1
  External Force and Torque5/RConn1 -- WFR/RConn1
  Simulink-PS Converter3/RConn1 -- External Force and Torque5/LConn5
  Simulink-PS Converter1/RConn1 -- External Force and Torque5/LConn4

== system WMMSupportingForcesGP2020a/Mobile Manipulator in Simscape/WRL_kinematic_quantities ==
  note: Friction momemnt and more to be added.
  FzRL_meas : Inport
  RL_kin : Inport  Port=2
  MyaRL : Inport  Port=3
  Bus Selector : BusSelector  OutputSignals=alphaRL_meas,dOmegaRL_meas,kappaRL_meas,ReRL,VxRL_meas
  Constant : Constant  Value=0
  External Force and Torque1 : sm_lib/Forces and Torques/External Force and Torque  ForceResolutionFrame=AttachedFrame  EnableForceX=off  EnableForceY=off  EnableForceZ=off  EnableForce=off  TorqueResolutionFrame=AttachedFrame  EnableTorqueX=off  EnableTorqueY=on  EnableTorqueZ=off  EnableTorque=off
  External Force and Torque5 : sm_lib/Forces and Torques/External Force and Torque  ForceResolutionFrame=AttachedFrame  EnableForceX=on  EnableForceY=on  EnableForceZ=on  EnableForce=off  TorqueResolutionFrame=AttachedFrame  EnableTorqueX=on  EnableTorqueY=on  EnableTorqueZ=off  EnableTorque=off
  Gain3 : Gain  Gain=1e4
  Gain6 : Gain  Gain=R0RL
  Gain7 : Gain  Gain=-R0RL
  Product : Product
  Product2 : Product
  Simulink-PS Converter{1..3,7,11,13} (6 alike) : nesl_utility/Simulink-PS Converter  PhysicalDomain=network_engine_domain  SubClassName=ps_input  LeftPortType=input  RightPortType=output  PseudoPeriodic=off  Frequencies=[]  NoiseDistribution=none  NoiseParameters=[]  Unit=1  AffineConversion=off  FilteringAndDerivatives=provide  SimscapeFilterOrder=1  InputFilterTimeConstant=0.001  UdotUserProvided=0
      settings: SourceProductBaseCode=PW,SS
  Sum2 : Sum  Inputs=-++
  Tanh : Trigonometry  Operator=tanh
  Terminator : Terminator
  lateralForceRL : MATLAB Function  TreatAsAtomicUnit=on
  longitudinalForceRL : MATLAB Function  TreatAsAtomicUnit=on
  WRL : PMIOPort  Side=Left
  WRLp : PMIOPort  Port=2  Side=Left
  wires:
  MyaRL/1 -> [MyaRL]
  [ReRL] -> Product/1
  [FzRL_meas] -> lateralForceRL/1(FzRL)
  Bus Selector/1 -> [alphaRL_meas]  "<alphaRL_meas>"
  [FzRL_meas] -> longitudinalForceRL/1(FzRL)
  Bus Selector/4 -> [ReRL]  "<ReRL>"
  Bus Selector/3 -> [kappaRL_meas]  "<kappaRL_meas>"
  Bus Selector/2 -> Terminator/1  "<dOmegaRL_meas>"
  FzRL_meas/1 -> [FzRL_meas]
  RL_kin/1 -> Bus Selector/1
  Sum2/1 -> Simulink-PS Converter2/1
  [FxRL] -> Product/2
  [MyaRL] -> Sum2/3
  [FxRL] -> Simulink-PS Converter13/1
  [FyRL] -> Simulink-PS Converter11/1
  [FzRL_meas] -> Simulink-PS Converter7/1
  Product/1 -> Sum2/1
  Constant/1 -> Sum2/2
  [FyRL] -> Gain6/1
  Gain6/1 -> Simulink-PS Converter1/1
  [FxRL] -> Gain7/1
  Gain7/1 -> Simulink-PS Converter3/1
  [VxRL_meas] -> Gain3/1
  Tanh/1 -> [sgnVxRL]
  Gain3/1 -> Tanh/1
  Product2/1 -> [FxRL]
  longitudinalForceRL/1(FxRL) -> Product2/2
  lateralForceRL/1(FyRL) -> [FyRL]
  [sgnVxRL] -> Product2/1
  Bus Selector/5 -> [VxRL_meas]  "<VxRL_meas>"
  [kappaRL_meas] -> longitudinalForceRL/2(kappaRL)
  [alphaRL_meas] -> lateralForceRL/2(alphaRL)
  connections:
  External Force and Torque5/RConn1 -- WRL/RConn1
  Simulink-PS Converter2/RConn1 -- External Force and Torque1/LConn1
  Simulink-PS Converter11/RConn1 -- External Force and Torque5/LConn2
  Simulink-PS Converter7/RConn1 -- External Force and Torque5/LConn3
  External Force and Torque1/RConn1 -- WRLp/RConn1
  Simulink-PS Converter13/RConn1 -- External Force and Torque5/LConn1
  Simulink-PS Converter3/RConn1 -- External Force and Torque5/LConn5
  Simulink-PS Converter1/RConn1 -- External Force and Torque5/LConn4

== system WMMSupportingForcesGP2020a/Mobile Manipulator in Simscape/WRR_kinematic_quantities ==
  note: Friction momemnt and more to be added.
  FzRR_meas : Inport
  RR_kin : Inport  Port=2
  MyaRR : Inport  Port=3
  Bus Selector : BusSelector  OutputSignals=alphaRR_meas,dOmegaRR_meas,kappaRR_meas,ReRR,VxRR_meas
  Constant : Constant  Value=0
  External Force and Torque1 : sm_lib/Forces and Torques/External Force and Torque  ForceResolutionFrame=AttachedFrame  EnableForceX=off  EnableForceY=off  EnableForceZ=off  EnableForce=off  TorqueResolutionFrame=AttachedFrame  EnableTorqueX=off  EnableTorqueY=on  EnableTorqueZ=off  EnableTorque=off
  External Force and Torque5 : sm_lib/Forces and Torques/External Force and Torque  ForceResolutionFrame=AttachedFrame  EnableForceX=on  EnableForceY=on  EnableForceZ=on  EnableForce=off  TorqueResolutionFrame=AttachedFrame  EnableTorqueX=on  EnableTorqueY=on  EnableTorqueZ=off  EnableTorque=off
  Gain2 : Gain  Gain=R0RR
  Gain5 : Gain  Gain=-R0RR
  Gain6 : Gain  Gain=1e4
  Product : Product
  Product2 : Product
  Simulink-PS Converter{1..3,7,11,13} (6 alike) : nesl_utility/Simulink-PS Converter  PhysicalDomain=network_engine_domain  SubClassName=ps_input  LeftPortType=input  RightPortType=output  PseudoPeriodic=off  Frequencies=[]  NoiseDistribution=none  NoiseParameters=[]  Unit=1  AffineConversion=off  FilteringAndDerivatives=provide  SimscapeFilterOrder=1  InputFilterTimeConstant=0.001  UdotUserProvided=0
      settings: SourceProductBaseCode=PW,SS
  Sum2 : Sum  Inputs=-++
  Tanh : Trigonometry  Operator=tanh
  Terminator : Terminator
  lateralForceRR : MATLAB Function  TreatAsAtomicUnit=on
  longitudinalForceRR : MATLAB Function  TreatAsAtomicUnit=on
  WRR : PMIOPort  Side=Left
  WRRp : PMIOPort  Port=2  Side=Left
  wires:
  MyaRR/1 -> [MyaRR]
  [ReRR] -> Product/1
  [FzRR_meas] -> lateralForceRR/1(FzRR)
  Bus Selector/1 -> [alphaRR_meas]  "<alphaRR_meas>"
  [FzRR_meas] -> longitudinalForceRR/1(FzRR)
  Bus Selector/4 -> [ReRR]  "<ReRR>"
  Bus Selector/3 -> [kappaRR_meas]  "<kappaRR_meas>"
  Bus Selector/2 -> Terminator/1  "<dOmegaRR_meas>"
  FzRR_meas/1 -> [FzRR_meas]
  RR_kin/1 -> Bus Selector/1
  Sum2/1 -> Simulink-PS Converter2/1
  [FxRR] -> Product/2
  [MyaRR] -> Sum2/3
  [FxRR] -> Simulink-PS Converter13/1
  [FyRR] -> Simulink-PS Converter11/1
  [FzRR_meas] -> Simulink-PS Converter7/1
  Product/1 -> Sum2/1
  Constant/1 -> Sum2/2
  Gain2/1 -> Simulink-PS Converter1/1
  [FyRR] -> Gain2/1
  [FxRR] -> Gain5/1
  Gain5/1 -> Simulink-PS Converter3/1
  lateralForceRR/1(FyRR) -> [FyRR]
  [sgnVxRR] -> Product2/1
  longitudinalForceRR/1(FxRR) -> Product2/2
  Product2/1 -> [FxRR]
  Bus Selector/5 -> [VxRR_meas]  "<VxRR_meas>"
  [kappaRR_meas] -> longitudinalForceRR/2(kappaRR)
  [alphaRR_meas] -> lateralForceRR/2(alphaRR)
  [VxRR_meas] -> Gain6/1
  Tanh/1 -> [sgnVxRR]
  Gain6/1 -> Tanh/1
  connections:
  External Force and Torque5/RConn1 -- WRR/RConn1
  Simulink-PS Converter2/RConn1 -- External Force and Torque1/LConn1
  Simulink-PS Converter11/RConn1 -- External Force and Torque5/LConn2
  Simulink-PS Converter7/RConn1 -- External Force and Torque5/LConn3
  External Force and Torque1/RConn1 -- WRRp/RConn1
  Simulink-PS Converter13/RConn1 -- External Force and Torque5/LConn1
  Simulink-PS Converter3/RConn1 -- External Force and Torque5/LConn5
  Simulink-PS Converter1/RConn1 -- External Force and Torque5/LConn4

== system WMMSupportingForcesGP2020a/Mobile Manipulator in Simscape/calc_VC_from_meas ==
  VCx_meas : Inport
  VCy_meas : Inport  Port=2
  Product6 : Product
  Product7 : Product
  Sqrt : Sqrt  SaturateOnIntegerOverflow=on
  Sum16 : Sum  Inputs=|++
  VC_meas : Outport
  wires:
  Product7/1 -> Sum16/2
  VCx_meas/1 -> Product6/1, Product6/2
  Product6/1 -> Sum16/1
  VCy_meas/1 -> Product7/1, Product7/2
  Sum16/1 -> Sqrt/1
  Sqrt/1 -> VC_meas/1

== system WMMSupportingForcesGP2020a/Mobile Manipulator in Simscape/calc_betaC_from_meas ==
  VCy_meas : Inport
  VCx_meas : Inport  Port=2
  meas_VFL1 : Subsystem
  betaC_meas : Outport
  wires:
  VCy_meas/1 -> [BCvy_meas]
  VCx_meas/1 -> [BCvx_meas]
  [betaC_meas] -> betaC_meas/1
  meas_VFL1/1(alphaFL_meas) -> [betaC_meas]
  [BCvy_meas] -> meas_VFL1/2(VFLy_meas)
  [BCvx_meas] -> meas_VFL1/1(VFLx_meas)
